simulink model "Rossler"  (R2019b)
settings: Solver=VariableStepAuto  StartTime=0.0  StopTime=10.0  RelTol=1e-3  EnableMultiTasking=on
undefined symbols (not defined in the file or in its folder): sfunxyz
settings Model: Creator=Elena  LastModifiedBy=Elena

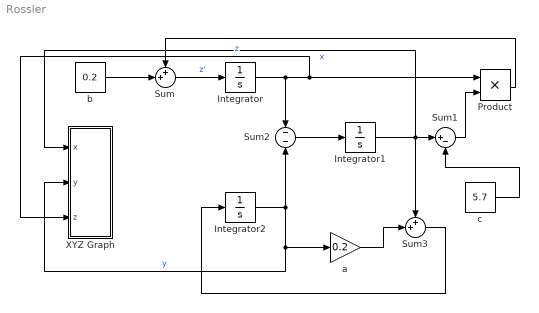
== system Rossler ==
  Integrator : Integrator
  Integrator1 : Integrator
  Integrator2 : Integrator
  Product : Product
  Sum : Sum  Inputs=++|
  Sum1 : Sum  Inputs=|+-
  Sum2 : Sum  Inputs=-|-
  Sum3 : Sum  Inputs=++|
  XYZ Graph : Subsystem  LoadFcn=sfunxyz([],[],[],'LoadBlock')  StartFcn=sfunxyz([],[],[],'Start')  StopFcn=sfunxyz([],[],[],'Stop')  mask(XYZ multiscope){np=2, xyzlim=[-50 50 -50 50 -50 50], cp=[50 49 48], gd=on, st=0.1}
      mask prompts: np "Number of lines"; xyzlim "[xmin xmax, ymin ymax, zmin zmax]"; cp "Camera position (use [0 0 1] for 2D XY view)"; gd "Grid"; st "Sample time:"
      mask help:
      | Multidimensional XYZ scope using MATLAB graph window.
      |    X,Y,Z coordinates are respectively the first,second, and third input.
      |    Enter the number of lines, the XYZ ranges, the camera position,
      |    and the sampling time, as mask parameters.
      settings: CopyFcn=sfunxyz([],[],[],'CopyBlock')  DeleteFcn=sfunxyz([],[],[],'DeleteBlock')  NameChangeFcn=sfunxyz([],[],[],'NameChange')
      mask Help:
      | This block can be used to explore limit cycles.
      |    Look at the m-file sfunxyz.m to see how it works.
      mask Display: plot([.05 .95 .95 .05 .05],[.45 .45 .95 .95 .45], 0.5+cos(0:0.1:2*pi)*0.3,0.7+sin(0:0.1:2*pi)*0.2)
  a : Gain  Gain=0.2
  "b " : Constant  Value=0.2
  c : Constant  Value=5.7
  wires:
  Sum3/1 -> Integrator2/1
  Sum2/1 -> Integrator1/1
  a/1 -> Sum3/2
  c/1 -> Sum1/2
  Integrator2/1 -> XYZ Graph/2(y), a/1, Sum2/2  "y"
  Product/1 -> Sum/1
  Sum1/1 -> Product/2
  Sum/1 -> Integrator/1  "z'"
  Integrator1/1 -> Sum3/1, XYZ Graph/1(x), Sum1/1  "x"
  "b "/1 -> Sum/2
  Integrator/1 -> XYZ Graph/3(z), Product/1, Sum2/1  "z"

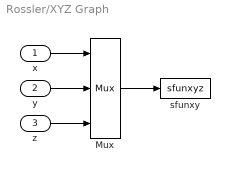
== system Rossler/XYZ Graph ==
  x : Inport
  y : Inport  Port=2
  z : Inport  Port=3
  Mux : Mux  Inputs=[np np np]
  sfunxy : S-Function  FunctionName=sfunxyz  Parameters=xyzlim,st,np,cp,gd  SFunctionDeploymentMode=off  EnableBusSupport=off
  wires:
  z/1 -> Mux/3
  y/1 -> Mux/2
  x/1 -> Mux/1
  Mux/1 -> sfunxy/1
